simulink model "mrac_pursuit_"  (R2020b)
settings: Solver=FixedStepAuto  StartTime=0.0  StopTime=T  FixedStep=0.01  RelTol=1e-3
values from neighbouring files (symbols this model uses):
  delay = params(2)    [integrator_delay.m]    (also in integrator_muscular_delay.m; mrac_model.m; mrac_model_e2y.m = params(4); mrac_model_e2y_2delay.m = params(6))
  gamma_r = 0.03    [cases_test.m]    (also in cases_tests_lr.m = gamma_r_0 * i; mrac_model_const_ref.m = params(6); mrac_model_lr.m = params(5); mrac_model_lr_init.m = params(8))
  gamma_x = [0.5; 0.5]    [cases_test.m]    (also in cases_tests_lr.m = gamma_x_0 * i; mrac_model_const_ref.m = params(4:5); mrac_model_e2y.m = params(5:6); mrac_model_e2y_2delay.m = params(7:8))
  k_r0 = k_r0_list(:, plant_case)    [cases_test.m]    (also in mrac_model_const_ref.m = params(3); mrac_model_lr_init.m = params(3); mrac_model_lr_init_low_pass.m = params(3); mrac_pursuit.m = params(3))
  k_x0 = k_x0_list(:, plant_case)    [cases_test.m]    (also in mrac_model_const_ref.m = [-params(1); params(2)]; mrac_model_e2y.m = params(1:2); mrac_model_e2y_2delay.m = params(1:2); mrac_model_lr_init.m = [-params(1); params(2)])
  P = lyap(ref_sys.A', eye(2))    [cases_test.m]    (also in cases_tests_lr.m; mrac_model_e2y.m = [1.5 1; 1.5, 1]; mrac_model_e2y_2delay.m = [1.5, 0; 1.5, 3.5]; mrac_model_lr_init_low_pass_comp.m = params(3:4))
  ref_sys = canon(ref_sys, 'modal')    [cases_test.m]    (also in cases_tests_lr.m; mrac_model.m = ss([tf_cl_pade; s*tf_cl_pade]); mrac_model_e2y.m = ss([tf_cl_pade; s*tf_cl_pade]); mrac_model_e2y_2delay.m = ss([tf_cl_pade; s*tf_cl_pade]))
undefined symbols (not defined in the file or in its folder): delay_model, dynamics_case, fast_transition, ref_x0, transition
settings Model: OrderedModelArguments=off  Creator=lorenzoterenzi  LastModifiedBy=lorenzoterenzi

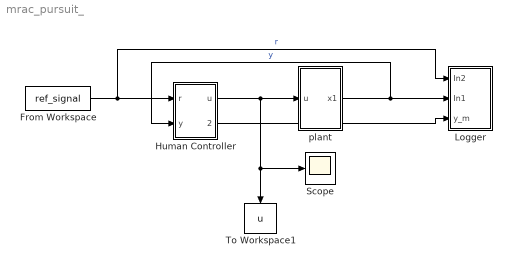
== system mrac_pursuit_ ==
  From Workspace : FromWorkspace  VariableName=ref_signal
  Human Controller : Subsystem
  Logger : Subsystem
  Scope : Scope
  To Workspace1 : ToWorkspace  VariableName=u  SaveFormat=Timeseries  SampleTime=-1
  plant : Subsystem
  wires:
  plant/1(x1) -> Human Controller/2(y), Logger/2(In1)  "y"
  From Workspace/1 -> Logger/1(In2), Human Controller/1(r)  "r"
  Human Controller/1(u) -> Scope/1, To Workspace1/1, plant/1(u)
  Human Controller/2(y_m) -> Logger/3(y_m)

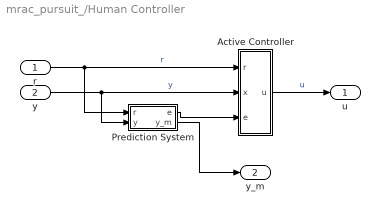
== system mrac_pursuit_/Human Controller ==
  r : Inport
  y : Inport  Port=2
  Active Controller : Subsystem
  Prediction System : Subsystem
  u : Outport
  y_m : Outport  Port=2
  wires:
  y/1 -> Active Controller/2(x), Prediction System/2(y)  "y"
  Active Controller/1(u) -> u/1  "u"
  r/1 -> Prediction System/1(r), Active Controller/1(r)  "r"
  Prediction System/1(e) -> Active Controller/3(e)
  Prediction System/2(y_m) -> y_m/1

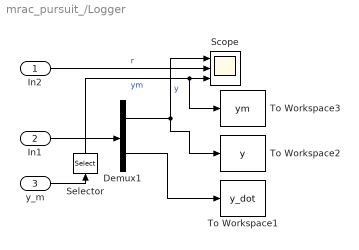
== system mrac_pursuit_/Logger ==
  In2 : Inport
  In1 : Inport  Port=2
  y_m : Inport  Port=3
  Demux1 : Demux  Outputs=2
  Scope : Scope  NumInputPorts=3
  Selector : Selector  InputPortWidth=2  IndexOptions=Index vector (dialog)  Indices=[1]  OutputSizes=1
  To Workspace1 : ToWorkspace  VariableName=y_dot  SaveFormat=Timeseries  SampleTime=-1
  To Workspace2 : ToWorkspace  VariableName=y  SaveFormat=Timeseries  SampleTime=-1
  To Workspace3 : ToWorkspace  VariableName=ym  SaveFormat=Timeseries  SampleTime=-1
  wires:
  In1/1 -> Demux1/1
  Demux1/2 -> To Workspace1/1
  Demux1/1 -> Scope/1, To Workspace2/1  "y"
  In2/1 -> Scope/2  "r"
  y_m/1 -> Selector/1
  Selector/1 -> To Workspace3/1, Scope/3  "ym"

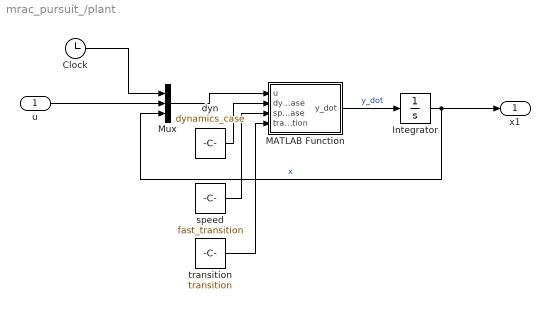
== system mrac_pursuit_/plant ==
  u : Inport
  Clock : Clock
  Integrator : Integrator  InitialCondition=[0;0]
  MATLAB Function : MATLAB Function  TreatAsAtomicUnit=on
  Mux : Mux  Inputs=3
  dyn : Constant  Value=dynamics_case
  speed : Constant  Value=fast_transition
  transition : Constant  Value=transition
  x1 : Outport
  wires:
  Mux/1 -> MATLAB Function/1(u)
  Integrator/1 -> x1/1, Mux/3  "x"
  MATLAB Function/1(y_dot) -> Integrator/1  "y_dot"
  Clock/1 -> Mux/1
  dyn/1 -> MATLAB Function/2(dynamics_case)
  u/1 -> Mux/2
  speed/1 -> MATLAB Function/3(speed_case)
  transition/1 -> MATLAB Function/4(transition)

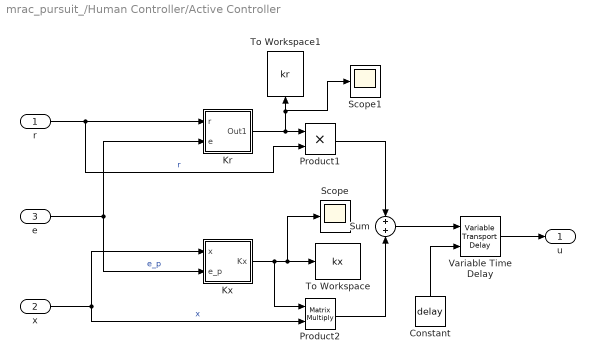
== system mrac_pursuit_/Human Controller/Active Controller ==
  r : Inport
  x : Inport  Port=2
  e : Inport  Port=3
  Constant : Constant  Value=delay
  Kr : Subsystem
  Kx : Subsystem
  Product1 : Product
  Product2 : Product  Multiplication=Matrix(*)
  Scope : Scope
  Scope1 : Scope
  Sum : Sum
  To Workspace : ToWorkspace  VariableName=kx  SaveFormat=Timeseries  SampleTime=-1
  To Workspace1 : ToWorkspace  VariableName=kr  SaveFormat=Timeseries  SampleTime=-1
  Variable Time Delay : VariableTransportDelay  MaximumDelay=10
  u : Outport
  wires:
  r/1 -> Product1/2, Kr/1(r)  "r"
  Product2/1 -> Sum/2
  Product1/1 -> Sum/1
  Kr/1(Out1) -> Product1/1, Scope1/1, To Workspace1/1
  e/1 -> Kx/2(e_p), Kr/2(e)  "e_p"
  x/1 -> Product2/2, Kx/1(x)  "x"
  Kx/1(Kx) -> Product2/1, Scope/1, To Workspace/1
  Sum/1 -> Variable Time Delay/1
  Variable Time Delay/1 -> u/1
  Constant/1 -> Variable Time Delay/2

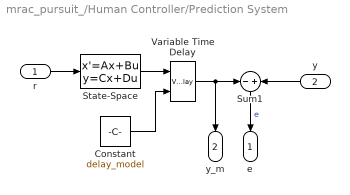
== system mrac_pursuit_/Human Controller/Prediction System ==
  r : Inport
  y : Inport  Port=2
  Constant : Constant  Value=delay_model
  State-Space : StateSpace  A=ref_sys.A  B=ref_sys.B  C=ref_sys.C  D=ref_sys.D  InitialCondition=ref_x0
  Sum1 : Sum  Inputs=-+
  Variable Time Delay : VariableTransportDelay  MaximumDelay=10
  e : Outport
  y_m : Outport  Port=2
  wires:
  Sum1/1 -> e/1  "e"
  r/1 -> State-Space/1
  y/1 -> Sum1/2
  State-Space/1 -> Variable Time Delay/1
  Variable Time Delay/1 -> y_m/1, Sum1/1
  Constant/1 -> Variable Time Delay/2

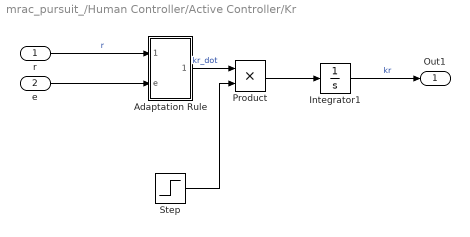
== system mrac_pursuit_/Human Controller/Active Controller/Kr ==
  r : Inport
  e : Inport  Port=2
  Adaptation Rule : Subsystem
  Integrator1 : Integrator  InitialCondition=k_r0
  Product : Product
  Step : Step  Time=0  SampleTime=0
  Out1 : Outport
  wires:
  Integrator1/1 -> Out1/1  "kr"
  r/1 -> Adaptation Rule/1(In1)  "r"
  e/1 -> Adaptation Rule/2(e)
  Adaptation Rule/1(Out1) -> Product/1  "kr_dot"
  Product/1 -> Integrator1/1
  Step/1 -> Product/2

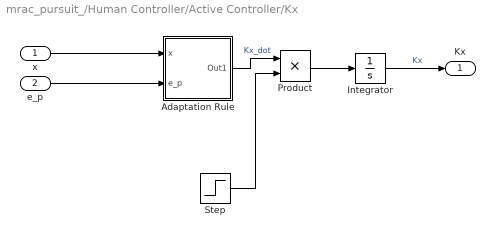
== system mrac_pursuit_/Human Controller/Active Controller/Kx ==
  x : Inport
  e_p : Inport  Port=2
  Adaptation Rule : Subsystem
  Integrator : Integrator  InitialCondition=k_x0
  Product : Product
  Step : Step  Time=0  SampleTime=0
  Kx : Outport
  wires:
  Integrator/1 -> Kx/1  "Kx"
  x/1 -> Adaptation Rule/1(x)
  e_p/1 -> Adaptation Rule/2(e_p)
  Adaptation Rule/1(Out1) -> Product/1  "Kx_dot"
  Product/1 -> Integrator/1
  Step/1 -> Product/2

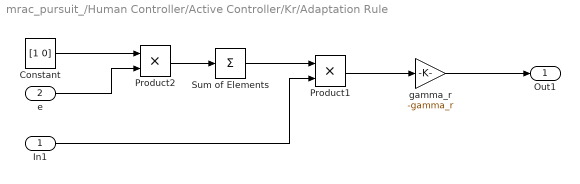
== system mrac_pursuit_/Human Controller/Active Controller/Kr/Adaptation Rule ==
  In1 : Inport
  e : Inport  Port=2
  Constant : Constant  Value=[1 0]
  Product1 : Product
  Product2 : Product
  Sum of Elements : Sum  Inputs=+
  gamma_r : Gain  Gain=-gamma_r
  Out1 : Outport
  wires:
  gamma_r/1 -> Out1/1
  Product2/1 -> Sum of Elements/1
  Constant/1 -> Product2/1
  e/1 -> Product2/2
  Product1/1 -> gamma_r/1
  Sum of Elements/1 -> Product1/1
  In1/1 -> Product1/2

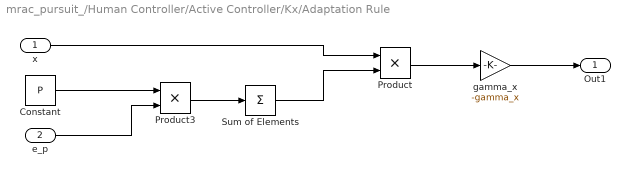
== system mrac_pursuit_/Human Controller/Active Controller/Kx/Adaptation Rule ==
  x : Inport
  e_p : Inport  Port=2
  Constant : Constant  Value=P
  Product : Product
  Product3 : Product
  Sum of Elements : Sum  Inputs=+
  gamma_x : Gain  Gain=-gamma_x
  Out1 : Outport
  wires:
  gamma_x/1 -> Out1/1
  x/1 -> Product/1
  Product3/1 -> Sum of Elements/1
  e_p/1 -> Product3/2
  Sum of Elements/1 -> Product/2
  Product/1 -> gamma_x/1
  Constant/1 -> Product3/1

== matlab function mrac_pursuit_/plant/MATLAB Function ==
  data: u input size=4; y_dot output size=2; dynamics_case input; speed_case input; transition input
function y_dot = fcn(u, dynamics_case, speed_case, transition)
    t = u(1);
    u_c = u(2);
    y_prev = u(3:4);
    
    if transition == 0
        y_dot = models.plant(dynamics_case, speed_case, t, u_c, y_prev);
    elseif transition == 1
        y_dot = models.plant_3_phases(dynamics_case, speed_case, t, u_c, y_prev);
    else 
        y_dot = [0;0];
    end
end


% function y_dot = peter_plant(case_, t, u, y_prev)
%     % case 1: first to second order system transition
%     if case_ == 1
%         M = -1;
%         G = -100;
%     % case 2: second to first order transition
%     elseif case_ == 2 
%         M = 91;
%         G = 100;
%     elseif case_ == 3    
%         M = 50;
%         G = 0.5;
%     elseif case_ == 4
%         M = 50;
%         G = 100;
%     else
%         G = 0;
%         M = 0;
%     end
% 
%     omega_b1 = 6;
%     omega_b2 = 0.2;
%     k_c1 = 90;
%     k_c2 = 30;
% 
%     omega_b = omega_b1 + (omega_b2 - omega_b1)./(1 + exp(-G * (t - M)));
%     k_c = k_c1 + (k_c2 - k_c1)./(1 + exp(-G * (t - M)));
% 
%     A = [0, 1; 0, omega_b];
%     B = [0; k_c];
%     y_dot = A*y_prev + B*u;
% end
